simulink model "simulation_scalar_exception"  (R2021b)
settings: Solver=VariableStepAuto  StartTime=0.0  StopTime=6  MaxStep=0.01  RelTol=1e-3
values from neighbouring files (symbols this model uses):
  k43 = 0    [exception.mat]    (also in robustness.mat = 663.324958071; scalar.mat = 61.6408497202; scalar_net.m = sqrt(2)*omega43*sqrt(abs(M(4,3)/M(3,4))); scalar_net_CreationNewConnection.m = sqrt(2)*omega43*sqrt(abs(M(4,3)/M(3,4))))
  k51 = 946.044396421    [exception.mat]    (also in robustness.mat = 146.385010942; scalar.mat = 259.670461528; scalar_net.m = sqrt(2)*omega51*sqrt(abs(M(5,1)/M(1,5))); scalar_net_CreationNewConnection.m = sqrt(2)*omega51*sqrt(abs(M(5,1)/M(1,5))))
  M = [-1.5 0 -0.7 0 17.9 0 -4.1 -6.8 0 0 0 0 ... (25 elements, 5x5)]    [exception.mat]    (also in nonscalar.mat = [-3.8 1.9 -4.5 0 0 0 -4.6 1.6 0 0 0 0 ... (25 elements, 5x5); nonscalar_net.m = round(M,1); nonscalar_net_general.m = sym('M',sum(n)); robustness.mat = [-8.5 0 -1.6 0 1.5 0 -5.3 -4.7 0 0 0 0 ... (25 elements, 5x5)
  omega43 = 50    [exception.mat]    (also in robustness.mat; scalar.mat; scalar_net.m = 200; scalar_net_CreationNewConnection.m)
  omega51 = 50    [exception.mat]    (also in robustness.mat = 70.7106781187; scalar.mat = 70.7106781187; scalar_net.m = sqrt(2) * omega_0; scalar_net_CreationNewConnection.m = sqrt(2) * omega_0)
  x_0 = [1 1 1 1 1]    [exception.mat]    (also in nonscalar_net.m = ones(sum(n),1); robustness.mat; scalar.mat; scalar_net.m = ones(5,1))
settings Model: Creator=alber  LastModifiedBy=anobili

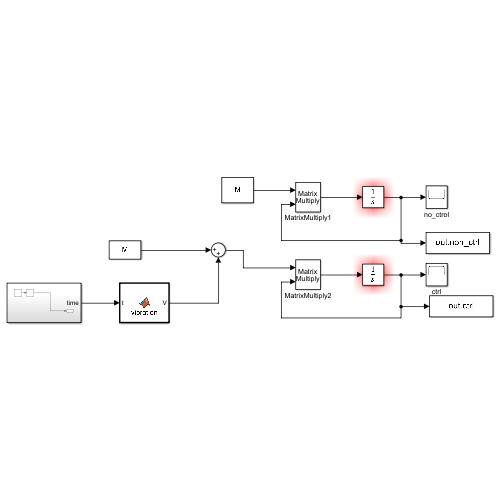
[thumbnail: Simulink's stored preview of the top-level diagram]
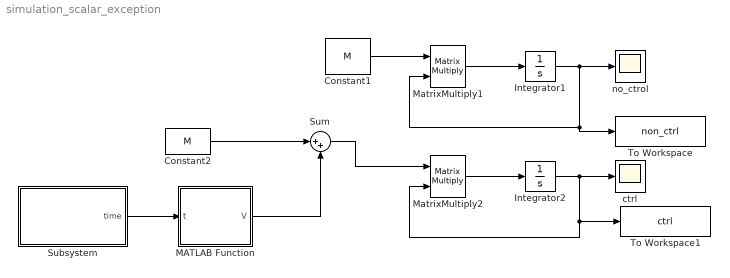
== system simulation_scalar_exception ==
  Constant1 : Constant  Value=M
  Constant2 : Constant  Value=M
  Integrator1 : Integrator  InitialCondition=x_0
  Integrator2 : Integrator  InitialCondition=x_0
  MATLAB Function : MATLAB Function  TreatAsAtomicUnit=on
  MatrixMultiply1 : Product  Multiplication=Matrix(*)
  MatrixMultiply2 : Product  Multiplication=Matrix(*)
  Subsystem : Subsystem
  Sum : Sum  Inputs=|++
  To Workspace : ToWorkspace  VariableName=non_ctrl  SaveFormat=Timeseries  SampleTime=-1
  To Workspace1 : ToWorkspace  VariableName=ctrl  SaveFormat=Timeseries  SampleTime=-1
  ctrl : Scope
  no_ctrol : Scope
  wires:
  MatrixMultiply1/1 -> Integrator1/1
  Constant1/1 -> MatrixMultiply1/1
  Integrator1/1 -> no_ctrol/1, To Workspace/1, MatrixMultiply1/2
  Constant2/1 -> Sum/1
  Integrator2/1 -> ctrl/1, To Workspace1/1, MatrixMultiply2/2
  MatrixMultiply2/1 -> Integrator2/1
  Sum/1 -> MatrixMultiply2/1
  Subsystem/1(time) -> MATLAB Function/1(t)
  MATLAB Function/1(V) -> Sum/2

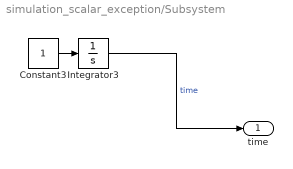
== system simulation_scalar_exception/Subsystem ==
  Constant3 : Constant
  Integrator3 : Integrator
  time : Outport
  wires:
  Constant3/1 -> Integrator3/1
  Integrator3/1 -> time/1  "time"

== matlab function simulation_scalar_exception/MATLAB Function ==
  data: t input; V output; omega43 parameter; k43 parameter; omega51 parameter; k51 parameter
function V = vibration(t, omega43, k43, omega51, k51)

V = zeros(5);
V(5,1) = k51*sin(omega51*t);
V(4,3) = k43*sin(omega43*t);
